simulink model "SDOF_SMD_input_PID"  (R2016a)
settings: Solver=FixedStepAuto  StartTime=0.0  StopTime=10.0  FixedStep=1/F_s  RelTol=1e-3
undefined symbols (not defined in the file): C, D, F_s, I, K, M, P
libraries: simulink x1
settings Model: Creator=ROB  LastModifiedBy=ROB

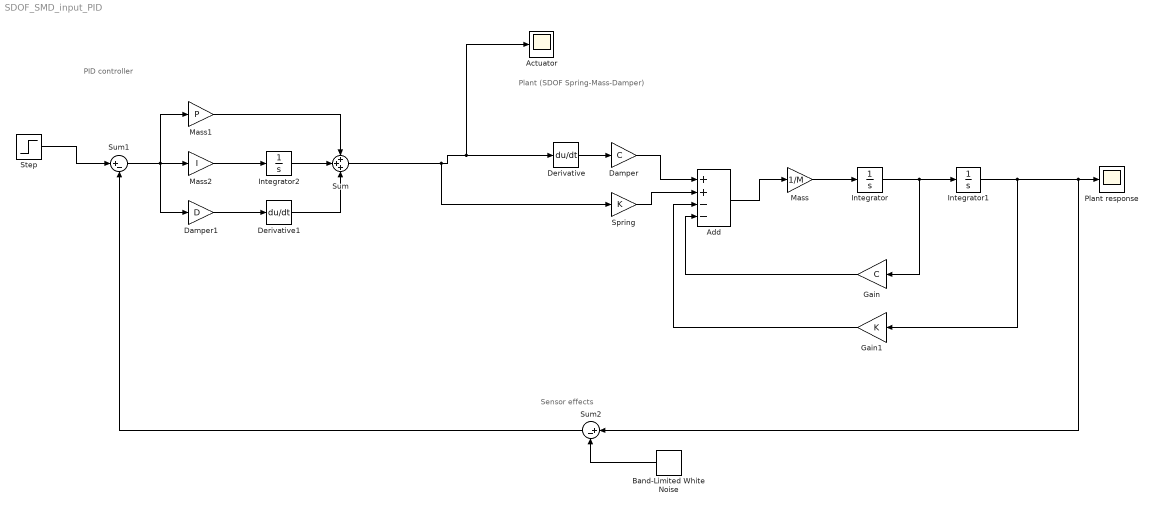
== system SDOF_SMD_input_PID ==
  note: Sensor effects
  note: PID controller
  note: Plant (SDOF Spring-Mass-Damper)
  Actuator : Scope
  Add : Sum  Inputs=++--
  Band-Limited White Noise : simulink/Sources/Band-Limited White Noise  Cov=[0.00001]  Ts=1/F_s  seed=[23341]
  Damper : Gain  Gain=C
  Damper1 : Gain  Gain=D
  Derivative : Derivative
  Derivative1 : Derivative
  Gain : Gain  Gain=C
  Gain1 : Gain  Gain=K
  Integrator : Integrator
  Integrator1 : Integrator
  Integrator2 : Integrator
  Mass : Gain  Gain=1/M
  Mass1 : Gain  Gain=P
  Mass2 : Gain  Gain=I
  "Plant response " : Scope
  "Spring " : Gain  Gain=K
  Step : Step  SampleTime=0
  Sum : Sum  Inputs=+++
  Sum1 : Sum  Inputs=|+-
  Sum2 : Sum  Inputs=|+-
  wires:
  Add/1 -> Mass/1
  Mass/1 -> Integrator/1
  Integrator/1 -> Gain/1, Integrator1/1
  Gain/1 -> Add/4
  Integrator1/1 -> Gain1/1, Sum2/1, "Plant response "/1
  Gain1/1 -> Add/3
  "Spring "/1 -> Add/2
  Derivative/1 -> Damper/1
  Damper/1 -> Add/1
  Damper1/1 -> Derivative1/1
  Mass2/1 -> Integrator2/1
  Integrator2/1 -> Sum/2
  Mass1/1 -> Sum/1
  Derivative1/1 -> Sum/3
  Sum/1 -> "Spring "/1, Actuator/1, Derivative/1
  Sum1/1 -> Damper1/1, Mass1/1, Mass2/1
  Step/1 -> Sum1/1
  Band-Limited White Noise/1 -> Sum2/2
  Sum2/1 -> Sum1/2
